simulink model "egr"  (Simulink 7.5)
settings: Solver=ode45  StartTime=0.0  StopTime=0.1  RelTol=1e-3
libraries: powerlib x23, powerlib_extras x2
settings Model: Creator=new user  LastModifiedBy=Administrator
settings DebuggingCC: StrictBusMsg=Warning

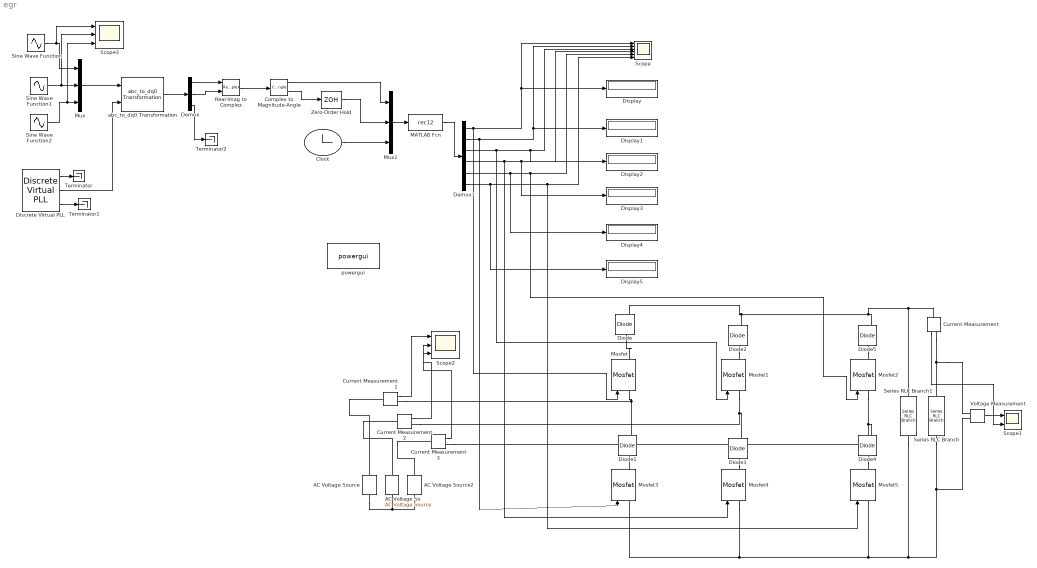
== system egr ==
  AC Voltage So : powerlib/Electrical Sources/AC Voltage Source  DialogController=POWERSYS.PowerSysDialog  SystemSampleTime=-1  Amplitude=230*sqrt(2)  Phase=120  Frequency=50  SampleTime=0  Measurements=None
  AC Voltage Source : powerlib/Electrical Sources/AC Voltage Source  DialogController=POWERSYS.PowerSysDialog  SystemSampleTime=-1  Amplitude=230*sqrt(2)  Phase=0  Frequency=50  SampleTime=0  Measurements=None
  AC Voltage Source2 : powerlib/Electrical Sources/AC Voltage Source  DialogController=POWERSYS.PowerSysDialog  SystemSampleTime=-1  Amplitude=230*sqrt(2)  Phase=-120  Frequency=50  SampleTime=0  Measurements=None
  Clock : Clock
  Complex to Magnitude-Angle : ComplexToMagnitudeAngle  SampleTime=2.5e-07
  Current Measurement{,1..3} (4 alike) : powerlib/Measurements/Current Measurement  DialogController=POWERSYS.PowerSysDialog  SystemSampleTime=-1  PhasorSimulation=off  OutputType=Complex  PSBequivalent=0
  Demux : Demux  Outputs=3
  Demux1 : Demux  Outputs=6
  Diode{,1..5} (6 alike) : powerlib/Power Electronics/Diode  DialogController=POWERSYS.PowerSysDialog  SystemSampleTime=-1  Ron=0.001  Lon=0  Vf=0.8  IC=0  UseSnubber=off  Rs=500  Cs=250e-9  Measurements=on
  Discrete Virtual PLL : powerlib_extras/Discrete  Control Blocks/Discrete Virtual PLL  DialogController=POWERSYS.PowerSysDialog  SystemSampleTime=-1  Freq=25  Phase=0  Ts=2.5e-07
  Display{,1..5} (6 alike) : Display
  MATLAB Fcn : MATLABFcn  MATLABFcn=rec12  OutputDimensions=6
  Mosfet{,1..5} (6 alike) : powerlib/Power Electronics/Mosfet  DialogController=POWERSYS.PowerSysDialog  SystemSampleTime=-1  Ron=0.1  Lon=0  Rd=0.01  Vfd=0  IC=0  Rs=1e5  Cs=inf  Measurements=on
  Mux : Mux  Inputs=3
  Mux1 : Mux  Inputs=3
  Real-Imag to Complex : RealImagToComplex  SampleTime=2.5e-07
  Scope : Scope  NumInputPorts=6
      settings: YMin=0~0~0~0~0~0  YMax=1~1~1~1~1~1
  Scope1 : Scope  NumInputPorts=2
      settings: YMin=512.5~20.5  YMax=555~22.2  SaveName=voltage
  Scope2 : Scope  NumInputPorts=3
      settings: YMin=-350~-300~-350  YMax=350~350~350
  Scope3 : Scope  NumInputPorts=3
      settings: YMin=0~175~-217  YMax=42.5~200~-199  SaveName=ScopeData3
  Series RLC Branch : powerlib/Elements/Series RLC Branch  DialogController=POWERSYS.PowerSysDialog  PhysicalDomain=powersysdomain  SubClassName=unknown  LeftPortType=p1  RightPortType=p1  LConnTagsString=__new0  RConnTagsString=__new0  BranchType=R  Resistance=25  Inductance=100e-3  SetiL0=off  InitialCurrent=0  Capacitance=1e-6  Setx0=off  InitialVoltage=0  Measurements=None
  Series RLC Branch1 : powerlib/Elements/Series RLC Branch  DialogController=POWERSYS.PowerSysDialog  PhysicalDomain=powersysdomain  SubClassName=unknown  LeftPortType=p1  RightPortType=p1  LConnTagsString=__new0  RConnTagsString=__new0  BranchType=Open circuit  Resistance=100  Inductance=40e-3  SetiL0=off  InitialCurrent=0  Capacitance=1000e-6  Setx0=off  InitialVoltage=0  Measurements=None
  Sine Wave Function : Sin  Amplitude=230  Bias=0  Frequency=2*pi*25  Phase=0  Samples=10  SampleTime=2.5e-07  Offset=0
  Sine Wave Function1 : Sin  Amplitude=230  Bias=0  Frequency=2*pi*25  Phase=2*pi/3  Samples=10  SampleTime=2.5e-07  Offset=0
  Sine Wave Function2 : Sin  Amplitude=230  Bias=0  Frequency=2*pi*25  Phase=4*pi/3  Samples=10  SampleTime=2.5e-07  Offset=0
  Terminator : Terminator
  Terminator1 : Terminator
  Terminator2 : Terminator
  Voltage Measurement : powerlib/Measurements/Voltage Measurement  DialogController=POWERSYS.PowerSysDialog  SystemSampleTime=-1  PhasorSimulation=off  OutputType=Complex  PSBequivalent=0
  Zero-Order Hold : ZeroOrderHold  SampleTime=.0001005
  abc_to_dq0 Transformation : powerlib_extras/Measurements/abc_to_dq0 Transformation  DialogController=POWERSYS.PowerSysDialog  SystemSampleTime=-1
  powergui : powerlib/powergui  Priority=1  SystemSampleTime=-1  SimulationMode=Discrete  SampleTime=2.5e-07  frequency=60  SPID=off  DisableSnubberDevices=off  DisableRonSwitches=off  DisableVfSwitches=off  SwTol=0  Interpol=off  frequencyindice=0  echomessages=off  HookPort=off  DisplayEquations=off  FunctionMessages=off  EnableUseOfTLC=off  x0status=blocks  RestoreLinks=warning  ResistiveCurrentMeasurement=off  Frange=[0:2:500]  Ylog=off  Xlog=on  ShowGrid=off  save=off  variable=ZData  structure=ScopeData1  ZoomFFT=off  StartTime=0.02  cycles=1  DisplayStyle=3  fundamental=50  FreqAxis=off  MaxFrequency=1000  frequencyindicesteady=0  RmsSteady=2  display=off  Ts=0  methode=off
  wires:
  Discrete Virtual PLL/1 -> Terminator/1
  Discrete Virtual PLL/3 -> Terminator1/1
  Sine Wave Function/1 -> Mux/1, Scope3/1
  Sine Wave Function1/1 -> Mux/2, Scope3/2
  Sine Wave Function2/1 -> Mux/3, Scope3/3
  Mux/1 -> abc_to_dq0 Transformation/1
  Discrete Virtual PLL/2 -> abc_to_dq0 Transformation/2
  abc_to_dq0 Transformation/1 -> Demux/1
  Demux/3 -> Terminator2/1
  Demux/1 -> Real-Imag to Complex/1
  Demux/2 -> Real-Imag to Complex/2
  Real-Imag to Complex/1 -> Complex to Magnitude-Angle/1
  Complex to Magnitude-Angle/2 -> Zero-Order Hold/1
  Complex to Magnitude-Angle/1 -> Mux1/1
  Zero-Order Hold/1 -> Mux1/2
  Mux1/1 -> MATLAB Fcn/1
  MATLAB Fcn/1 -> Demux1/1
  Demux1/1 -> Scope/1, Display/1, Mosfet/1
  Demux1/2 -> Scope/2, Display1/1, Mosfet3/1
  Demux1/3 -> Scope/3, Display2/1, Mosfet1/1
  Demux1/4 -> Scope/4, Display3/1, Mosfet4/1
  Demux1/5 -> Display4/1, Scope/5, Mosfet2/1
  Demux1/6 -> Display5/1, Scope/6, Mosfet5/1
  Voltage Measurement/1 -> Scope1/1
  Clock/1 -> Mux1/3
  Current Measurement/1 -> Scope1/2
  Current Measurement1/1 -> Scope2/1
  Current Measurement2/1 -> Scope2/2
  Current Measurement3/1 -> Scope2/3
  connections:
  Voltage Measurement/LConn1 -- Series RLC Branch/LConn1 -- Current Measurement/RConn1
  Series RLC Branch/RConn1 -- Voltage Measurement/LConn2 -- Mosfet5/LConn1 -- Mosfet4/LConn1 -- Mosfet3/LConn1 -- Series RLC Branch1/RConn1
  AC Voltage Source/LConn1 -- AC Voltage Source2/LConn1 -- AC Voltage So/LConn1
  Current Measurement/LConn1 -- Series RLC Branch1/LConn1 -- Diode/RConn1 -- Diode2/RConn1 -- Diode5/RConn1
  Diode/LConn1 -- Mosfet/RConn1
  Mosfet3/RConn1 -- Diode1/LConn1
  Diode2/LConn1 -- Mosfet1/RConn1
  Diode3/LConn1 -- Mosfet4/RConn1
  Diode4/LConn1 -- Mosfet5/RConn1
  Diode5/LConn1 -- Mosfet2/RConn1
  Mosfet/LConn1 -- Diode1/RConn1 -- Current Measurement1/RConn1
  Mosfet1/LConn1 -- Diode3/RConn1 -- Current Measurement2/RConn1
  Mosfet2/LConn1 -- Diode4/RConn1 -- Current Measurement3/RConn1
  AC Voltage Source/RConn1 -- Current Measurement1/LConn1
  AC Voltage So/RConn1 -- Current Measurement2/LConn1
  AC Voltage Source2/RConn1 -- Current Measurement3/LConn1
